simulink model "LandinModel"  (R2020a)
settings: Solver=ode1  StartTime=0.0  StopTime=100  FixedStep=0.05  RelTol=1e-3
values from neighbouring files (symbols this model uses):
  BMV_Spring_Constant = spring_constant    [run_monte_carlo.m]
  Pedal_Angular_Displacement = 9    [run_monte_carlo.m]
  Pedal_Force = 50    [run_monte_carlo.m]
undefined symbols (not defined in the file or in its folder): AC_d, Air_Density, Airplane_Mass, Brake_Friction_Coefficient, Engine_Thrust, Landing_Velocity, Rolling_Friction_Coefficient, Runway_Downslope
libraries: BrakeSystemLibrary x1
settings Model: Creator=Jared  LastModifiedBy=Jared

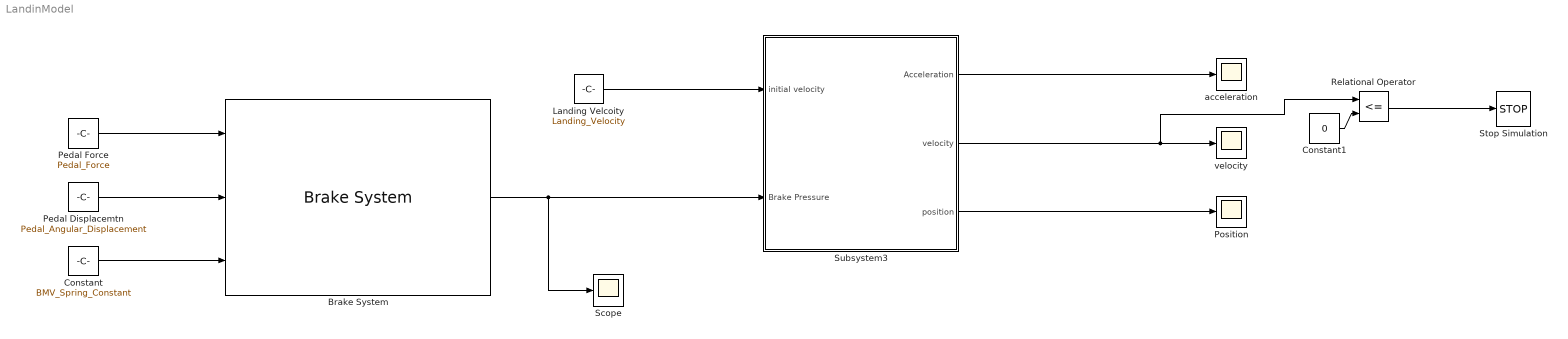
== system LandinModel ==
  Brake System : BrakeSystemLibrary/Brake System  SystemSampleTime=-1  Latency=0  AutoFrameSizeCalculation=off
  Constant : Constant  Value=BMV_Spring_Constant
  Constant1 : Constant  Value=0
  Landing Velcoity : Constant  Value=Landing_Velocity
  Pedal Displacemtn : Constant  Value=Pedal_Angular_Displacement
  Pedal Force : Constant  Value=Pedal_Force
  Position : Scope
  Relational Operator : RelationalOperator  Operator=<=  OutDataTypeStr=boolean  RndMeth=Simplest
  Scope : Scope
  Stop Simulation : Stop
  Subsystem3 : Subsystem
  acceleration : Scope
  velocity : Scope
  wires:
  Pedal Displacemtn/1 -> Brake System/2
  Pedal Force/1 -> Brake System/1
  Constant/1 -> Brake System/3
  Subsystem3/1(Acceleration) -> acceleration/1
  Subsystem3/2(velocity) -> Relational Operator/1, velocity/1
  Subsystem3/3(position) -> Position/1
  Landing Velcoity/1 -> Subsystem3/1(initial velocity)
  Relational Operator/1 -> Stop Simulation/1
  Constant1/1 -> Relational Operator/2
  Brake System/1 -> Scope/1, Subsystem3/2(Brake Pressure)

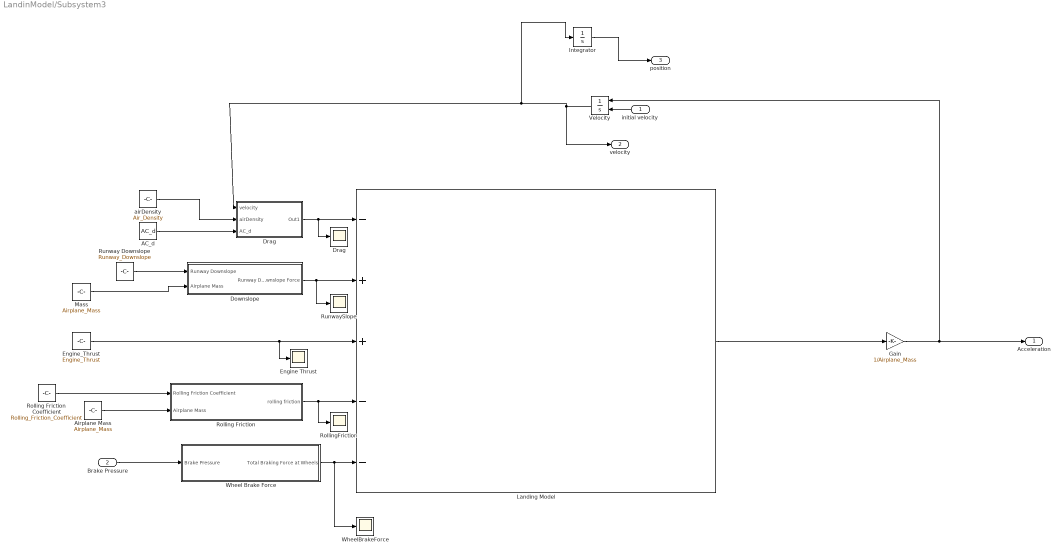
== system LandinModel/Subsystem3 ==
  initial velocity : Inport
  Brake Pressure : Inport  Port=2
  AC_d : Constant  Value=AC_d
  Airplane Mass : Constant  Value=Airplane_Mass
  Downslope : Subsystem
  Drag : Scope
  "Drag   " : Subsystem
  Engine Thrust : Scope
  Engine_Thrust : Constant  Value=Engine_Thrust
  Gain : Gain  Gain=1/Airplane_Mass
  Integrator : Integrator
  Landing Model : Sum  Inputs=-++--
  Mass : Constant  Value=Airplane_Mass
  Rolling Friction : Subsystem
  Rolling Friction Coefficient : Constant  Value=Rolling_Friction_Coefficient
  RollingFriction : Scope
  Runway Downslope : Constant  Value=Runway_Downslope
  RunwaySlope : Scope
  Velocity : Integrator  InitialConditionSource=external
  Wheel Brake Force : Subsystem
  WheelBrakeForce : Scope
  airDensity : Constant  Value=Air_Density
  Acceleration : Outport
  velocity : Outport  Port=2
  position : Outport  Port=3
  wires:
  Airplane Mass/1 -> Rolling Friction/2(Airplane Mass)
  Integrator/1 -> position/1
  Rolling Friction/1(rolling friction) -> RollingFriction/1, Landing Model/4
  Brake Pressure/1 -> Wheel Brake Force/1(Brake Pressure)
  "Drag   "/1(Out1) -> Drag/1, Landing Model/1
  Gain/1 -> Acceleration/1, Velocity/1
  Downslope/1(Runway Downslope Force) -> RunwaySlope/1, Landing Model/2
  airDensity/1 -> "Drag   "/2(airDensity)
  Velocity/1 -> Integrator/1, "Drag   "/1(velocity), velocity/1
  Mass/1 -> Downslope/2(Airplane Mass)
  Runway Downslope/1 -> Downslope/1(Runway Downslope)
  Landing Model/1 -> Gain/1
  Rolling Friction Coefficient/1 -> Rolling Friction/1(Rolling Friction Coefficient)
  Engine_Thrust/1 -> Engine Thrust/1, Landing Model/3
  Wheel Brake Force/1(Total Braking Force at Wheels) -> WheelBrakeForce/1, Landing Model/5
  AC_d/1 -> "Drag   "/3(AC_d)
  initial velocity/1 -> Velocity/2

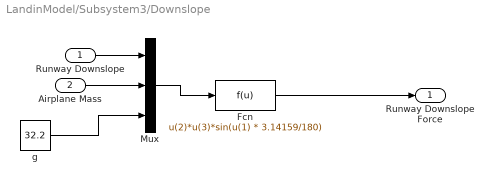
== system LandinModel/Subsystem3/Downslope ==
  Runway Downslope : Inport
  Airplane Mass : Inport  Port=2
  Fcn : Fcn  Expr=u(2)*u(3)*sin(u(1) * 3.14159/180)
  Mux : Mux  Inputs=3
  g : Constant  Value=32.2
  Runway Downslope Force : Outport
  wires:
  Fcn/1 -> Runway Downslope Force/1
  Mux/1 -> Fcn/1
  Runway Downslope/1 -> Mux/1
  Airplane Mass/1 -> Mux/2
  g/1 -> Mux/3

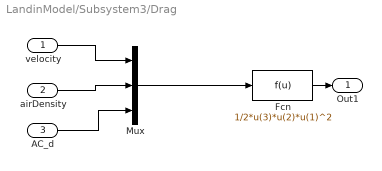
== system LandinModel/Subsystem3/Drag    ==
  velocity : Inport
  airDensity : Inport  Port=2
  AC_d : Inport  Port=3
  Fcn : Fcn  Expr=1/2*u(3)*u(2)*u(1)^2
  Mux : Mux  Inputs=3
  Out1 : Outport
  wires:
  velocity/1 -> Mux/1
  airDensity/1 -> Mux/2
  Mux/1 -> Fcn/1
  AC_d/1 -> Mux/3
  Fcn/1 -> Out1/1

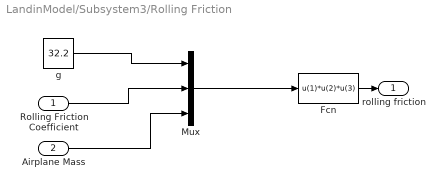
== system LandinModel/Subsystem3/Rolling Friction ==
  Rolling Friction Coefficient : Inport
  Airplane Mass : Inport  Port=2
  Fcn : Fcn  Expr=u(1)*u(2)*u(3)
  Mux : Mux  Inputs=3
  g : Constant  Value=32.2
  rolling friction : Outport
  wires:
  Airplane Mass/1 -> Mux/3
  g/1 -> Mux/1
  Rolling Friction Coefficient/1 -> Mux/2
  Mux/1 -> Fcn/1
  Fcn/1 -> rolling friction/1

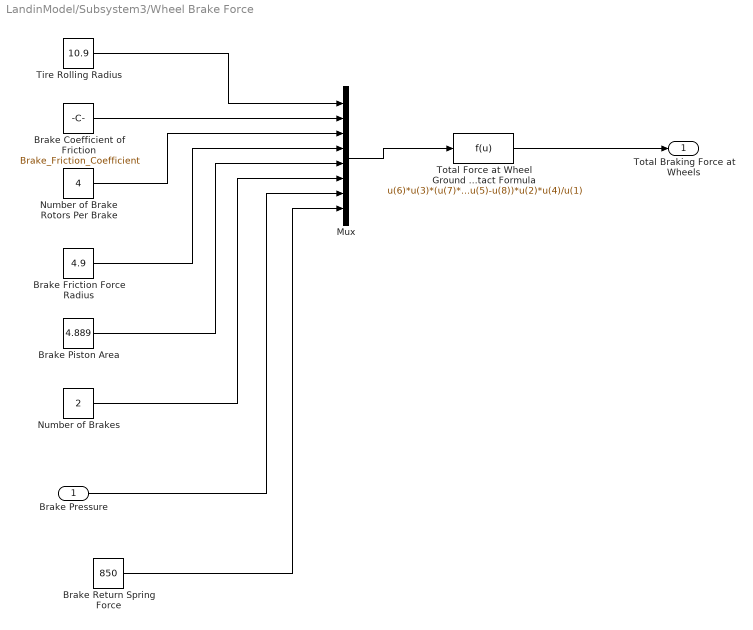
== system LandinModel/Subsystem3/Wheel Brake Force ==
  Brake Pressure : Inport
  Brake Coefficient of Friction : Constant  Value=Brake_Friction_Coefficient
  Brake Friction Force Radius : Constant  Value=4.9
  Brake Piston Area : Constant  Value=4.889
  Brake Return Spring Force : Constant  Value=850
  Mux : Mux  Inputs=8
  Number of Brake Rotors Per Brake : Constant  Value=4
  Number of Brakes : Constant  Value=2
  Tire Rolling Radius : Constant  Value=10.9
  Total Force at Wheel Ground Contact Formula : Fcn  Expr=u(6)*u(3)*(u(7)*u(5)-u(8))*u(2)*u(4)/u(1)
  Total Braking Force at Wheels : Outport
  wires:
  Brake Friction Force Radius/1 -> Mux/4
  Number of Brakes/1 -> Mux/6
  Brake Coefficient of Friction/1 -> Mux/2
  Brake Pressure/1 -> Mux/7
  Total Force at Wheel Ground Contact Formula/1 -> Total Braking Force at Wheels/1
  Tire Rolling Radius/1 -> Mux/1
  Brake Piston Area/1 -> Mux/5
  Mux/1 -> Total Force at Wheel Ground Contact Formula/1
  Number of Brake Rotors Per Brake/1 -> Mux/3
  Brake Return Spring Force/1 -> Mux/8
